simulink model "CarModel"  (R2016a)
settings: Solver=VariableStepAuto  StartTime=0  StopTime=3.1  MaxStep=0.3  RelTol=1e-5
values from neighbouring files (symbols this model uses):
  initialVelocity = 25.0    [CarDict.sldd]    (also in CarDict2.sldd = 20.0
  pressureGain = 1000000.0    [CarDict.sldd]    (also in CarDict2.sldd = 1800000.0
  rollingRadius = 0.3    [CarDict.sldd]    (also in CarDict2.sldd)
libraries: fl_lib x26, nesl_utility x14, sdl_lib x11, simulink x2
settings Model: DataDictionary=CarDict.sldd  FPTRunName=FPA_Reference  PauseTimes=3  Creator=oskar  LastModifiedBy=oskar
settings SolverCC: AlgebraicLoopSolver=LineSearch  SolverResetMethod=Robust
settings DataIOCC: SaveFormat=StructureWithTime  ReturnWorkspaceOutputs=on  ReturnWorkspaceOutputsName=spidata
settings HardwareCC: ProdBitPerLong=64  ProdLargestAtomicFloat=None  ProdHWDeviceType=Intel->x86-64  TargetBitPerLong=64  TargetBitPerPointer=64  TargetIntDivRoundTo=Zero  TargetEndianess=LittleEndian  TargetWordSize=64  TargetHWDeviceType=Intel->x86-64
settings RTWCC: SystemTargetFile=sldrt.tlc  TemplateMakefile=sldrt.tmf  Description=Simulink Desktop Real-Time  RTWCompilerOptimization=on  CheckMdlBeforeBuild=Error
settings CodeAppCC: MaxIdLength=95
settings SimulinkDesktopRealTimeCC: TargetPreCompLibLocation=/Applications/MATLAB_R2016a.app/toolbox/sldrt/lib/maci64  TargetLangStandard=C89/C90 (ANSI)  CodeReplacementLibrary=GNU C99 extensions  SupportVariableSizeSignals=off
settings SimscapeCC: SimscapeLogSimulationStatistics=on  SimscapeLogLimitData=off

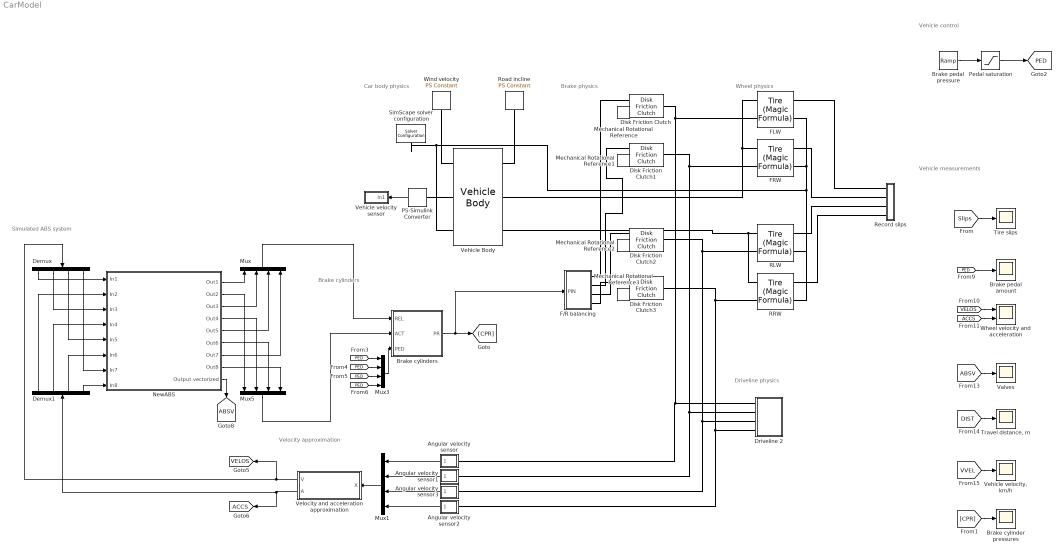
== system CarModel ==
  note: Velocity approximation
  note: Driveline physics
  note: Wheel physics
  note: Brake physics
  note: Car body physics
  note: Simulated ABS system
  note: Brake cylinders
  note: Vehicle control
  note: Vehicle measurements
  Angular velocity sensor : Subsystem
  Angular velocity sensor1 : Subsystem
  Angular velocity sensor2 : Subsystem
  Angular velocity sensor3 : Subsystem
  Brake cylinders : Subsystem  TreatAsAtomicUnit=on  mask(Brake cylinder){ABSGain=5.25, smooth=1e-2}
      mask prompts: ABSGain "ABS valve gain"; smooth "Smoothness"
      mask help:
      | A simple approximation of a brake cylinder w. pressure and relief valve inputs from the ABS system. The applied brake pressure is applied by the signal input on the port PED (symbolizing pressure from the master cylinder, or brake pedal). ACT and REL symbolize the pressure and relief valve inputs, respectively. All input values should be in the range [0,1], where 0 is no pressure and 1 maximum pressure.
      |
      | The system is tuned by the ABS gain parameter which scales the input of the ABS valves, and thus controlling the effeciency of those valves. The smoothing parameter regulates the smoothness of the pressure changes. The system outputs brake pressure in the range [0,10e5] Pa.
  Brake cylinder pressures : Scope
  Brake pedal pressure : simulink/Sources/Ramp  slope=5  start=0.5  X0=0
  Brake pedal amount : Scope
  Demux : Demux
  Demux1 : Demux
  Disk Friction Clutch{,1..3} (4 alike) : sdl_lib/Clutches/Disk Friction Clutch  geometry_model=1  r_eff=torqueRadius mm  d_o=150 mm  d_i=100 mm  nS=numSurf  piston_area=pistonArea m^2  unidirectional=0  friction_model=1  mu_coulomb=clutchKineticF  mu_w_vector=[ 0 0.1 0.2 0.3 0.4 0.5 1 2 5 10 100 1000 ] rad/s  mu_coulomb_vector=[ 0.29 0.28 0.26 0.22 0.21 0.2 0.2 0.19 0.19 0.19 0.19 0.19 ]  mu_interp_method=1  mu_extrap_method=1  mu_static=clutchStaticF  d_f=1  w_tol=clutchVeloTolRads rad/s  pressure_min=clutchPressureTresh Pa  mu_visc=0 N*m/(rad/s)  initial_state_locked=0
  Driveline 2 : Subsystem
  F/R balancing : Subsystem  mask(F/R Balance){RGain=0.5}
      mask prompts: RGain "Rear pressure gain"
      mask help: Scale the amount of pressure directed to the rear wheels by a constant factor (default 0.7).
  FLW : sdl_lib/Tires & Vehicles/Tire (Magic Formula)  parameterization=1  F_z1=2.5e+3 N  F_x1=3.5e+3 N  kappa1=10  B_m=10  C_m=1.9  D_m=1  E_m=0.97  fz0=4e+3 N  p_Cx=1.685  p_Dx=[ 1.21 -0.037 ]  p_Ex=[ 0.344 0.095 -0.02 0 ]  p_Kx=[ 21.51 -0.163 0.245 ]  p_Hx=[ -0.002 0.002 ]  p_Vx=[ 0 0 ]  v_tr_thr=0.1 m/s  r_e=rollingRadius m  model_compliance=0  stiffness=1e+6 N/m  damping=1000 N/(m/s)  model_inertia=0  inertia=1 kg*m^2  initial_velocity=0 rad/s  model_resistance=0  resistance_model=1  coeff=0.015  p_tire=250e3 Pa  alpha=-0.003  beta=0.97  coeff_a=84e-4  coeff_b=6.2e-4 s/m  coeff_c=1.6e-4 s^2/m^2  v_thr=1e-3 m/s
  FRW : sdl_lib/Tires & Vehicles/Tire (Magic Formula)  parameterization=1  F_z1=3e+3 N  F_x1=3.5e+3 N  kappa1=10  B_m=10  C_m=1.9  D_m=1  E_m=0.97  fz0=4e+3 N  p_Cx=1.685  p_Dx=[ 1.21 -0.037 ]  p_Ex=[ 0.344 0.095 -0.02 0 ]  p_Kx=[ 21.51 -0.163 0.245 ]  p_Hx=[ -0.002 0.002 ]  p_Vx=[ 0 0 ]  v_tr_thr=0.1 m/s  r_e=rollingRadius m  model_compliance=0  stiffness=1e+6 N/m  damping=1000 N/(m/s)  model_inertia=0  inertia=1 kg*m^2  initial_velocity=0 rad/s  model_resistance=0  resistance_model=1  coeff=0.015  p_tire=250e3 Pa  alpha=-0.003  beta=0.97  coeff_a=84e-4  coeff_b=6.2e-4 s/m  coeff_c=1.6e-4 s^2/m^2  v_thr=1e-3 m/s
  Mechanical Rotational Reference{,1..3} (4 alike) : fl_lib/Mechanical/Rotational Elements/Mechanical Rotational Reference
  Mux{,1,3,5} (4 alike) : Mux
  NewABS : Subsystem  mask(ARSim){simPath='/Users/oskar/dev/autosar/NewABS/dist/build/NewABSExt/NewABSExt', numInput=8, numOutput=8}
      mask prompts: simPath "Simulator path"; numInput "# input ports"; numOutput "# output ports"
      mask help:
      | This component acts as an S-function wrapper for the ARSim component. The simulator path parameter needs to be configured as a string pointing to the location of the compiled AUTOSAR component (i.e. with simulateUsingExternal).
      |
      | When the model is initialized, the AUTOSAR simulator will ask for specific port widths. This cannot be adjusted automatically by the Simulink component (yet), so manual intervention is needed, hence the # input/output ports dialogs.
      mask Display: ;port_label('input', 1, 'VELO1');port_label('input', 2, 'ACCEL1');port_label('input', 3, 'VELO2');port_label('input', 4, 'ACCEL2');port_label('input', 5, 'VELO3');port_label('input', 6, 'ACCEL3');port_label('input', 7, 'VELO4');port_label('input', 8, 'ACCEL4');port_label('output', 1, 'RE1');port_label('output', 2, 'PR1');port_label('output', 3, 'RE2');port_label('output', 4, 'PR2');port_label('output', 5, 'RE3');port_label('output', 6, 'PR3');port_label('output', 7, 'RE4');port_label('output', 8, 'PR4')
  PS-Simulink Converter : nesl_utility/PS-Simulink Converter  PhysicalDomain=network_engine_domain  SubClassName=ps_output  LeftPortType=input  RightPortType=output  PseudoPeriodic=off  Frequencies=[]  Unit=m/s  AffineConversion=off
  Pedal saturation : Saturate  UpperLimit=1  OutDataTypeStr=Inherit: Inherit via back propagation
  RLW : sdl_lib/Tires & Vehicles/Tire (Magic Formula)  parameterization=1  F_z1=3e+3 N  F_x1=3.5e+3 N  kappa1=10  B_m=10  C_m=1.9  D_m=1  E_m=0.97  fz0=4e+3 N  p_Cx=1.685  p_Dx=[ 1.21 -0.037 ]  p_Ex=[ 0.344 0.095 -0.02 0 ]  p_Kx=[ 21.51 -0.163 0.245 ]  p_Hx=[ -0.002 0.002 ]  p_Vx=[ 0 0 ]  v_tr_thr=0.1 m/s  r_e=rollingRadius m  model_compliance=0  stiffness=1e+6 N/m  damping=1000 N/(m/s)  model_inertia=0  inertia=1 kg*m^2  initial_velocity=0 rad/s  model_resistance=0  resistance_model=1  coeff=0.015  p_tire=250e3 Pa  alpha=-0.003  beta=0.97  coeff_a=84e-4  coeff_b=6.2e-4 s/m  coeff_c=1.6e-4 s^2/m^2  v_thr=1e-3 m/s
  RRW : sdl_lib/Tires & Vehicles/Tire (Magic Formula)  parameterization=1  F_z1=3e+3 N  F_x1=3.5e+3 N  kappa1=10  B_m=10  C_m=1.9  D_m=1  E_m=0.97  fz0=4e+3 N  p_Cx=1.685  p_Dx=[ 1.21 -0.037 ]  p_Ex=[ 0.344 0.095 -0.02 0 ]  p_Kx=[ 21.51 -0.163 0.245 ]  p_Hx=[ -0.002 0.002 ]  p_Vx=[ 0 0 ]  v_tr_thr=0.1 m/s  r_e=rollingRadius m  model_compliance=0  stiffness=1e+6 N/m  damping=1000 N/(m/s)  model_inertia=0  inertia=1 kg*m^2  initial_velocity=0 rad/s  model_resistance=0  resistance_model=1  coeff=0.015  p_tire=250e3 Pa  alpha=-0.003  beta=0.97  coeff_a=84e-4  coeff_b=6.2e-4 s/m  coeff_c=1.6e-4 s^2/m^2  v_thr=1e-3 m/s
  Record slips : Subsystem
  Road incline : fl_lib/Physical Signals/Sources/PS Constant  constant=0
  SimScape solver configuration : nesl_utility/Solver Configuration  PhysicalDomain=network_engine_domain  SubClassName=solver  LeftPortType=input  RightPortType=generic  Accelerate=off  Tones=[]  Harmonics=[]  SimulateNoise=off  Profile=off  UseLocalSampling=off  EnableSwitchedLinearOptims=on  FrequencyDomain=off  UseCCode=off  RelTol=0.001  AbsTol=1e-06  MinStep=1e-09  ToWorkspace=off  RevertToSquareIcSolve=off  NumHomotopyIterations=100  PhasorMode=off  PhasorModeNumHarmonics=1  OverrideAbsTol=off  DoDC=off  ResidualTolerance=1e-09  UseLocalSolver=off  LocalSolverChoice=NE_TRAPEZOIDAL_ADVANCER  LocalSolverSampleTime=0.001  DoFixedCost=off  MaxNonlinIter=3  MaxModeIter=2  LinearAlgebra=Sparse  DelaysMemoryBudget=1024  AutomaticFiltering=on  FilteringTimeConstant=0.001
  Tire slips : Scope
  "Travel distance, m" : Scope
  Valves : Scope
  Vehicle velocity sensor : Subsystem
  "Vehicle velocity, km/h" : Scope
  Vehicle Body : sdl_lib/Tires & Vehicles/Vehicle Body  mass=1500 kg  n_w=2  x_f=1.4 m  x_r=1.6 m  y_c=0.5 m  area=3 m^2  Cd=0.4  v0=initialVelocity m/s
  Velocity and acceleration approximation : Subsystem  TreatAsAtomicUnit=on  mask(Velocity and acceleration approximation){varAdj=1/100}
      mask prompts: varAdj "Adjustment factor"
      mask help: Measures angular velocity of the wheel axis and approximates acceleration through a discrete derivative set to a time interval of 0.001. The adjustment factor converts the magnitude of the acceleration to something which the NewABS-controller expects, since the pressure- and relief sequencers generate pulses proportional to acceleration.
  Wheel velocity and acceleration : Scope  NumInputPorts=2
  Wind velocity : fl_lib/Physical Signals/Sources/PS Constant  constant=5
  tag scope: ABSV=global, ACCS=global, PED=global, VELOS=global
  wires:
  Brake pedal pressure/1 -> Pedal saturation/1
  Angular velocity sensor/1(Out1) -> Mux1/1
  Angular velocity sensor1/1(Out1) -> Mux1/2
  Angular velocity sensor3/1(Out1) -> Mux1/3
  Angular velocity sensor2/1(Out1) -> Mux1/4
  Mux1/1 -> Velocity and acceleration approximation/1(X)
  Mux3/1 -> Brake cylinders/3(PED)
  [Slips] -> Tire slips/1
  NewABS/7(Out7) -> Mux/4
  NewABS/5(Out5) -> Mux/3
  NewABS/1(Out1) -> Mux/1
  NewABS/3(Out3) -> Mux/2
  Pedal saturation/1 -> [PED]
  [PED] -> Mux3/1
  [PED] -> Mux3/2
  [PED] -> Mux3/3
  [PED] -> Mux3/4
  [PED] -> Brake pedal amount/1
  [VELOS] -> Wheel velocity and acceleration/1
  [ACCS] -> Wheel velocity and acceleration/2
  [ABSV] -> Valves/1
  NewABS/9(Output vectorized) -> [ABSV]
  PS-Simulink Converter/1 -> Vehicle velocity sensor/1(In1)
  [DIST] -> "Travel distance, m"/1
  [VVEL] -> "Vehicle velocity, km/h"/1
  [CPR] -> Brake cylinder pressures/1
  Brake cylinders/1(PR) -> F/R balancing/1(PIN), [CPR]
  Mux/1 -> Brake cylinders/1(REL)
  Mux5/1 -> Brake cylinders/2(ACT)
  NewABS/2(Out2) -> Mux5/1
  NewABS/4(Out4) -> Mux5/2
  NewABS/6(Out6) -> Mux5/3
  NewABS/8(Out8) -> Mux5/4
  Velocity and acceleration approximation/1(V) -> Demux/1, [VELOS]
  Velocity and acceleration approximation/2(A) -> Demux1/1, [ACCS]
  Demux1/1 -> NewABS/2(In2)
  Demux/1 -> NewABS/1(In1)
  Demux/2 -> NewABS/3(In3)
  Demux/3 -> NewABS/5(In5)
  Demux/4 -> NewABS/7(In7)
  Demux1/2 -> NewABS/4(In4)
  Demux1/3 -> NewABS/6(In6)
  Demux1/4 -> NewABS/8(In8)
  connections:
  Vehicle Body/RConn1 -- RRW/LConn1 -- RLW/LConn1
  Vehicle Body/RConn2 -- FLW/LConn1 -- FRW/LConn1
  Wind velocity/RConn1 -- Vehicle Body/LConn3
  Vehicle Body/LConn1 -- RLW/RConn2 -- RRW/RConn2 -- FLW/RConn2 -- FRW/RConn2 -- SimScape solver configuration/RConn1
  Road incline/RConn1 -- Vehicle Body/RConn3
  Driveline 2/LConn3 -- Angular velocity sensor3/LConn1 -- RLW/LConn2 -- Disk Friction Clutch2/RConn1
  PS-Simulink Converter/LConn1 -- Vehicle Body/LConn2
  Driveline 2/LConn2 -- Disk Friction Clutch1/RConn1 -- FRW/LConn2 -- Angular velocity sensor1/LConn1
  Driveline 2/LConn1 -- Angular velocity sensor/LConn1 -- Disk Friction Clutch/RConn1 -- FLW/LConn2
  Driveline 2/LConn4 -- Angular velocity sensor2/LConn1 -- RRW/LConn2 -- Disk Friction Clutch3/RConn1
  FLW/RConn1 -- Record slips/LConn1
  FRW/RConn1 -- Record slips/LConn2
  RLW/RConn1 -- Record slips/LConn3
  RRW/RConn1 -- Record slips/LConn4
  Mechanical Rotational Reference/LConn1 -- Disk Friction Clutch/LConn2
  Mechanical Rotational Reference1/LConn1 -- Disk Friction Clutch1/LConn2
  Mechanical Rotational Reference2/LConn1 -- Disk Friction Clutch2/LConn2
  Mechanical Rotational Reference3/LConn1 -- Disk Friction Clutch3/LConn2
  Disk Friction Clutch/LConn1 -- F/R balancing/RConn1
  Disk Friction Clutch1/LConn1 -- F/R balancing/RConn2
  Disk Friction Clutch2/LConn1 -- F/R balancing/RConn3
  Disk Friction Clutch3/LConn1 -- F/R balancing/RConn4

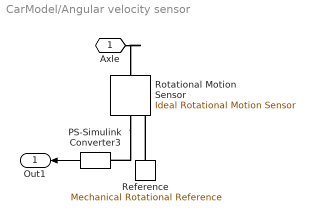
== system CarModel/Angular velocity sensor ==
  PS-Simulink Converter3 : nesl_utility/PS-Simulink Converter  PhysicalDomain=network_engine_domain  SubClassName=ps_output  LeftPortType=input  RightPortType=output  PseudoPeriodic=off  Frequencies=[]  Unit=rpm  AffineConversion=off
  Reference : fl_lib/Mechanical/Rotational Elements/Mechanical Rotational Reference
  Rotational Motion Sensor : fl_lib/Mechanical/Mechanical Sensors/Ideal Rotational Motion Sensor  offset=0 rad
  Axle : PMIOPort  Port=1  Side=Left
  Out1 : Outport
  wires:
  PS-Simulink Converter3/1 -> Out1/1
  connections:
  Axle/RConn1 -- Rotational Motion Sensor/LConn1
  Reference/LConn1 -- Rotational Motion Sensor/RConn1
  Rotational Motion Sensor/RConn2 -- PS-Simulink Converter3/LConn1

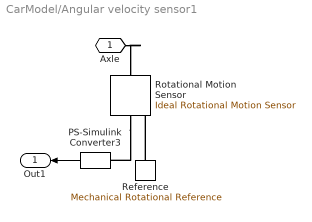
== system CarModel/Angular velocity sensor1 ==
  PS-Simulink Converter3 : nesl_utility/PS-Simulink Converter  PhysicalDomain=network_engine_domain  SubClassName=ps_output  LeftPortType=input  RightPortType=output  PseudoPeriodic=off  Frequencies=[]  Unit=rpm  AffineConversion=off
  Reference : fl_lib/Mechanical/Rotational Elements/Mechanical Rotational Reference
  Rotational Motion Sensor : fl_lib/Mechanical/Mechanical Sensors/Ideal Rotational Motion Sensor  offset=0 rad
  Axle : PMIOPort  Port=1  Side=Left
  Out1 : Outport
  wires:
  PS-Simulink Converter3/1 -> Out1/1
  connections:
  Axle/RConn1 -- Rotational Motion Sensor/LConn1
  Reference/LConn1 -- Rotational Motion Sensor/RConn1
  Rotational Motion Sensor/RConn2 -- PS-Simulink Converter3/LConn1

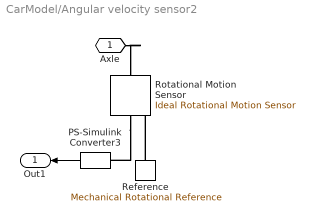
== system CarModel/Angular velocity sensor2 ==
  PS-Simulink Converter3 : nesl_utility/PS-Simulink Converter  PhysicalDomain=network_engine_domain  SubClassName=ps_output  LeftPortType=input  RightPortType=output  PseudoPeriodic=off  Frequencies=[]  Unit=rpm  AffineConversion=off
  Reference : fl_lib/Mechanical/Rotational Elements/Mechanical Rotational Reference
  Rotational Motion Sensor : fl_lib/Mechanical/Mechanical Sensors/Ideal Rotational Motion Sensor  offset=0 rad
  Axle : PMIOPort  Port=1  Side=Left
  Out1 : Outport
  wires:
  PS-Simulink Converter3/1 -> Out1/1
  connections:
  Axle/RConn1 -- Rotational Motion Sensor/LConn1
  Reference/LConn1 -- Rotational Motion Sensor/RConn1
  Rotational Motion Sensor/RConn2 -- PS-Simulink Converter3/LConn1

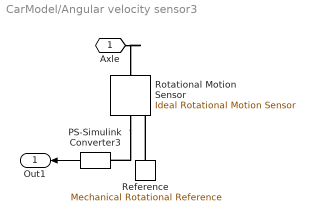
== system CarModel/Angular velocity sensor3 ==
  PS-Simulink Converter3 : nesl_utility/PS-Simulink Converter  PhysicalDomain=network_engine_domain  SubClassName=ps_output  LeftPortType=input  RightPortType=output  PseudoPeriodic=off  Frequencies=[]  Unit=rpm  AffineConversion=off
  Reference : fl_lib/Mechanical/Rotational Elements/Mechanical Rotational Reference
  Rotational Motion Sensor : fl_lib/Mechanical/Mechanical Sensors/Ideal Rotational Motion Sensor  offset=0 rad
  Axle : PMIOPort  Port=1  Side=Left
  Out1 : Outport
  wires:
  PS-Simulink Converter3/1 -> Out1/1
  connections:
  Axle/RConn1 -- Rotational Motion Sensor/LConn1
  Reference/LConn1 -- Rotational Motion Sensor/RConn1
  Rotational Motion Sensor/RConn2 -- PS-Simulink Converter3/LConn1

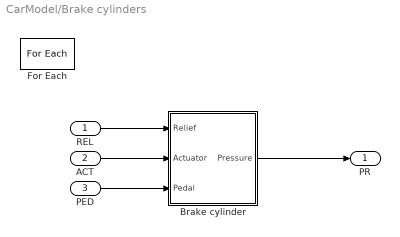
== system CarModel/Brake cylinders ==
  REL : Inport  Partition=on  PartitionDimension=1  PartitionWidth=1
  ACT : Inport  Port=2  Partition=on  PartitionDimension=1  PartitionWidth=1
  PED : Inport  Port=3  Partition=on  PartitionDimension=1  PartitionWidth=1
  Brake cylinder : Subsystem
  For Each : ForEach  DisableCoverage=on  IndexMode=One-based
  PR : Outport  Unit=Pa  ConcatenationDimension=1
  wires:
  PED/1 -> Brake cylinder/3(Pedal)
  ACT/1 -> Brake cylinder/2(Actuator)
  REL/1 -> Brake cylinder/1(Relief)
  Brake cylinder/1(Pressure) -> PR/1

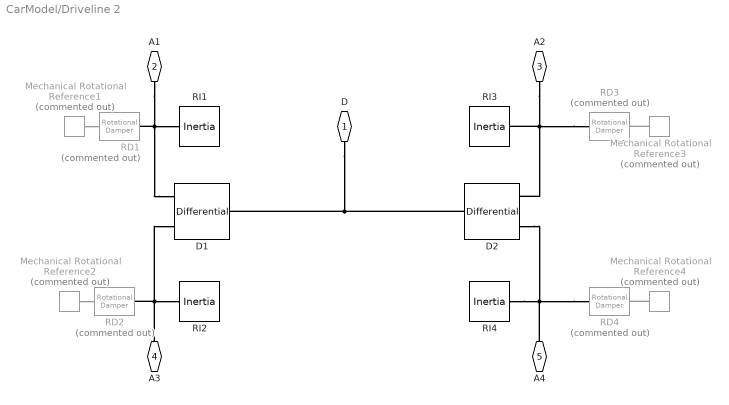
== system CarModel/Driveline 2 ==
  D1 : sdl_lib/Gears/Differential  driveshaft_location=2  cd_ratio=1  friction_model=1  efficiency=[ 0.85 0.92 ]  mu_visc=[ 0 0 ] N*m/(rad/s)  pwr_thr=[ 0.001 0.001 ] W  carrier_inertia=0 kg*m^2  planet_inertia=0 kg*m^2  temperature_TLU=[ 280 300 320 ] K  efficiency_ss_TLU=[ 0.95 0.9 0.85 ]  efficiency_cd_TLU=[ 0.95 0.9 0.85 ]  thermal_mass=50 J/K  T_init=300 K
  D2 : sdl_lib/Gears/Differential  driveshaft_location=2  cd_ratio=1  friction_model=1  efficiency=[ 0.85 0.92 ]  mu_visc=[ 0 0 ] N*m/(rad/s)  pwr_thr=[ 0.001 0.001 ] W  carrier_inertia=0 kg*m^2  planet_inertia=0 kg*m^2  temperature_TLU=[ 280 300 320 ] K  efficiency_ss_TLU=[ 0.95 0.9 0.85 ]  efficiency_cd_TLU=[ 0.95 0.9 0.85 ]  thermal_mass=50 J/K  T_init=300 K
  Mechanical Rotational Reference{1..4} (4 alike) : fl_lib/Mechanical/Rotational Elements/Mechanical Rotational Reference  Commented=on
  RD{1..4} (4 alike) : fl_lib/Mechanical/Rotational Elements/Rotational Damper  Commented=on  D=0.01 N*m/(rad/s)  w_specify=off  w_priority=High  w=0 rad/s  t_specify=off  t_priority=High  t=0 N*m
  RI{1..4} (4 alike) : fl_lib/Mechanical/Rotational Elements/Inertia  inertia=axleInertia kg*m^2  w_specify=on  w_priority=High  w=initialVelocity/rollingRadius rad/s  t_specify=off  t_priority=High  t=0 N*m
  D : PMIOPort  Port=1  Side=Right
  A1 : PMIOPort  Port=2  Side=Left
  A2 : PMIOPort  Port=3  Side=Left
  A3 : PMIOPort  Port=4  Side=Left
  A4 : PMIOPort  Port=5  Side=Left
  connections:
  Mechanical Rotational Reference1/LConn1 -- RD1/RConn1
  Mechanical Rotational Reference2/LConn1 -- RD2/RConn1
  Mechanical Rotational Reference3/LConn1 -- RD3/RConn1
  Mechanical Rotational Reference4/LConn1 -- RD4/RConn1
  D2/LConn1 -- D/RConn1 -- D1/LConn1
  RD4/LConn1 -- RI4/LConn1 -- D2/RConn2 -- A4/RConn1
  D1/RConn1 -- RI1/LConn1 -- A1/RConn1 -- RD1/LConn1
  RD3/LConn1 -- RI3/LConn1 -- D2/RConn1 -- A2/RConn1
  RD2/LConn1 -- RI2/LConn1 -- A3/RConn1 -- D1/RConn2

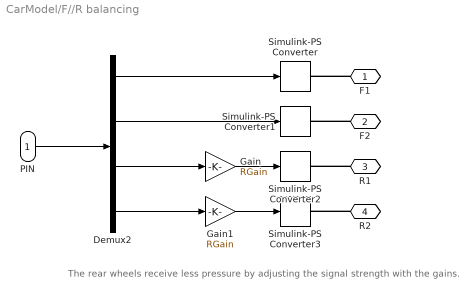
== system CarModel/F//R balancing ==
  note: The rear wheels receive less pressure by adjusting the signal strength with the gains.
  PIN : Inport
  Demux2 : Demux
  Gain : Gain  Gain=RGain
  Gain1 : Gain  Gain=RGain
  Simulink-PS Converter{,1..3} (4 alike) : nesl_utility/Simulink-PS Converter  PhysicalDomain=network_engine_domain  SubClassName=ps_input  LeftPortType=input  RightPortType=output  PseudoPeriodic=off  Frequencies=[]  NoiseDistribution=none  NoiseParameters=[]  Unit=Pa  AffineConversion=off  InputFiltering=off  SimscapeFilterOrder=1  InputFilterTimeConstant=0.001  UdotUserProvided=1
  F1 : PMIOPort  Port=1  Side=Right
  F2 : PMIOPort  Port=2  Side=Right
  R1 : PMIOPort  Port=3  Side=Right
  R2 : PMIOPort  Port=4  Side=Right
  wires:
  PIN/1 -> Demux2/1
  Demux2/1 -> Simulink-PS Converter/1
  Demux2/2 -> Simulink-PS Converter1/1
  Demux2/3 -> Gain/1
  Demux2/4 -> Gain1/1
  Gain/1 -> Simulink-PS Converter2/1
  Gain1/1 -> Simulink-PS Converter3/1
  connections:
  F1/RConn1 -- Simulink-PS Converter/RConn1
  F2/RConn1 -- Simulink-PS Converter1/RConn1
  R1/RConn1 -- Simulink-PS Converter2/RConn1
  R2/RConn1 -- Simulink-PS Converter3/RConn1

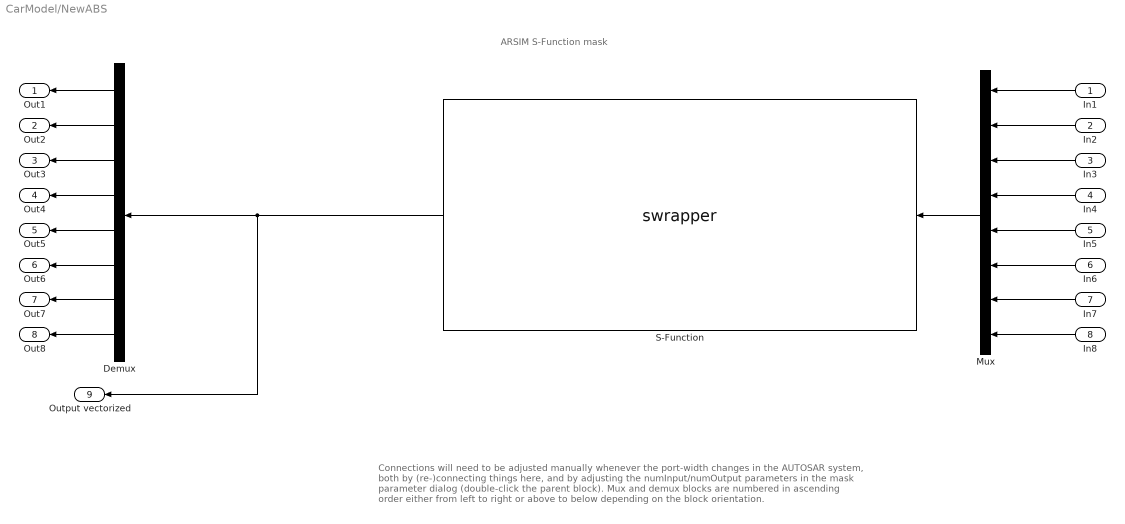
== system CarModel/NewABS ==
  note: ARSIM S-Function mask
  note: Connections will need to be adjusted manually whenever the port-width changes in the AUTOSAR system,
      | both by (re-)connecting things here, and by adjusting the numInput/numOutput parameters in the mask
      | parameter dialog (double-click the parent block).
      |
      | Mux and demux blocks are numbered in ascending order either from left to right or above to below depending
      | on the block orientation.
  In1 : Inport
  In2 : Inport  Port=2
  In3 : Inport  Port=3
  In4 : Inport  Port=4
  In5 : Inport  Port=5
  In6 : Inport  Port=6
  In7 : Inport  Port=7
  In8 : Inport  Port=8
  Demux : Demux  Outputs=numOutput
  Mux : Mux  Inputs=numInput
  S-Function : S-Function  FunctionName=swrapper  Parameters=simPath  SFunctionDeploymentMode=off  EnableBusSupport=off
  Out1 : Outport
  Out2 : Outport  Port=2
  Out3 : Outport  Port=3
  Out4 : Outport  Port=4
  Out5 : Outport  Port=5
  Out6 : Outport  Port=6
  Out7 : Outport  Port=7
  Out8 : Outport  Port=8
  Output vectorized : Outport  Port=9
  wires:
  In7/1 -> Mux/7
  In3/1 -> Mux/3
  In1/1 -> Mux/1
  In2/1 -> Mux/2
  In6/1 -> Mux/6
  In4/1 -> Mux/4
  In5/1 -> Mux/5
  In8/1 -> Mux/8
  Mux/1 -> S-Function/1
  S-Function/1 -> Output vectorized/1, Demux/1
  Demux/8 -> Out8/1
  Demux/7 -> Out7/1
  Demux/6 -> Out6/1
  Demux/5 -> Out5/1
  Demux/4 -> Out4/1
  Demux/3 -> Out3/1
  Demux/2 -> Out2/1
  Demux/1 -> Out1/1

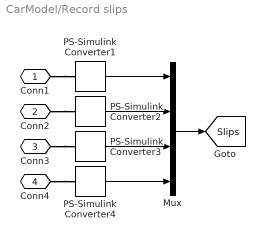
== system CarModel/Record slips ==
  Mux : Mux
  PS-Simulink Converter{1..4} (4 alike) : nesl_utility/PS-Simulink Converter  PhysicalDomain=network_engine_domain  SubClassName=ps_output  LeftPortType=input  RightPortType=output  PseudoPeriodic=off  Frequencies=[]  Unit=1  AffineConversion=off
  Conn1 : PMIOPort  Port=1  Side=Left
  Conn2 : PMIOPort  Port=2  Side=Left
  Conn3 : PMIOPort  Port=3  Side=Left
  Conn4 : PMIOPort  Port=4  Side=Left
  tag scope: Slips=global
  wires:
  Mux/1 -> [Slips]
  PS-Simulink Converter1/1 -> Mux/1
  PS-Simulink Converter2/1 -> Mux/2
  PS-Simulink Converter3/1 -> Mux/3
  PS-Simulink Converter4/1 -> Mux/4
  connections:
  Conn1/RConn1 -- PS-Simulink Converter1/LConn1
  Conn2/RConn1 -- PS-Simulink Converter2/LConn1
  Conn3/RConn1 -- PS-Simulink Converter3/LConn1
  Conn4/RConn1 -- PS-Simulink Converter4/LConn1

== system CarModel/Vehicle velocity sensor ==
  In1 : Inport  Unit=m/s
  Gain : Gain  Gain=3.6
  Integrator : Integrator
  tag scope: DIST=global, VVEL=global
  wires:
  In1/1 -> Integrator/1, Gain/1
  Gain/1 -> [VVEL]
  Integrator/1 -> [DIST]

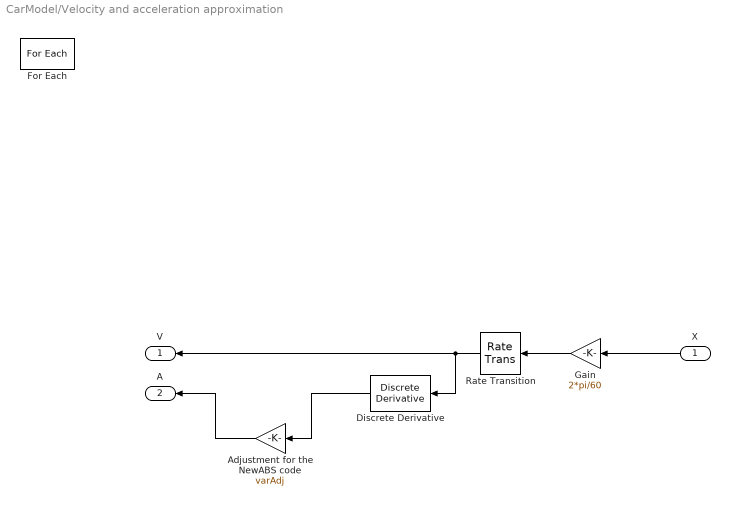
== system CarModel/Velocity and acceleration approximation ==
  X : Inport  Partition=on  PartitionDimension=1  PartitionWidth=1
  Adjustment for the NewABS code : Gain  Gain=varAdj
  Discrete Derivative : simulink/Discrete/Discrete Derivative  gainval=1  ICPrevScaledInput=0.0  OutMin=[]  OutMax=[]  OutDataType=fixdt(1, 16)  OutScaling=2^-10  DoSatur=off
  For Each : ForEach  DisableCoverage=on  IndexMode=One-based
  Gain : Gain  Gain=2*pi/60
  Rate Transition : RateTransition  OutPortSampleTime=0.001
  V : Outport  Unit=rad/s  ConcatenationDimension=1
  A : Outport  Port=2  Unit=rad/s/s  ConcatenationDimension=1
  wires:
  Rate Transition/1 -> V/1, Discrete Derivative/1
  Discrete Derivative/1 -> Adjustment for the NewABS code/1
  Gain/1 -> Rate Transition/1
  X/1 -> Gain/1
  Adjustment for the NewABS code/1 -> A/1

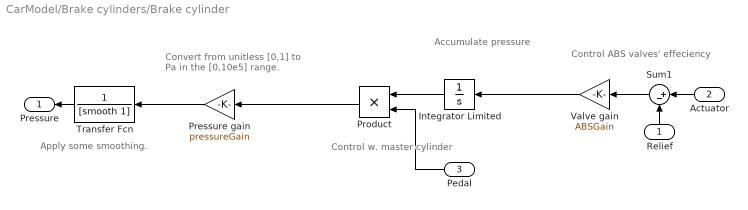
== system CarModel/Brake cylinders/Brake cylinder ==
  note: Apply some smoothing.
  note: Control ABS valves'
      | effeciency
  note: Control w.
      | master cylinder
  note: Accumulate
      | pressure
  note: Convert from unitless [0,1] to
      | Pa in the [0,10e5] range.
  Relief : Inport
  Actuator : Inport  Port=2
  Pedal : Inport  Port=3
  Integrator Limited : Integrator  LimitOutput=on  UpperSaturationLimit=1  LowerSaturationLimit=0
  Pressure gain : Gain  Gain=pressureGain
  Product : Product
  Sum1 : Sum  Inputs=|+-
  Transfer Fcn : TransferFcn  Denominator=[smooth 1]
  Valve gain : Gain  Gain=ABSGain
  Pressure : Outport
  wires:
  Actuator/1 -> Sum1/1
  Pressure gain/1 -> Transfer Fcn/1
  Relief/1 -> Sum1/2
  Integrator Limited/1 -> Product/1
  Product/1 -> Pressure gain/1
  Pedal/1 -> Product/2
  Valve gain/1 -> Integrator Limited/1
  Sum1/1 -> Valve gain/1
  Transfer Fcn/1 -> Pressure/1
